simulink model "Funcion_de_Costo"  (R2018b)
settings: Solver=VariableStepAuto  StartTime=0.0  StopTime=10.0  RelTol=1e-3
undefined symbols (not defined in the file or in its folder): DiscIntNeverNeededParam
settings Model: Creator=of  LastModifiedBy=of

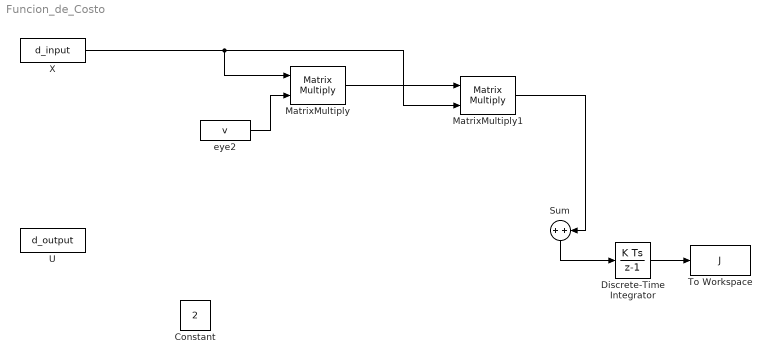
== system Funcion_de_Costo ==
  Constant : Constant  Value=2
  Discrete-Time Integrator : DiscreteIntegrator  SampleTime=-1  ICPrevOutput=DiscIntNeverNeededParam  ICPrevScaledInput=DiscIntNeverNeededParam
  MatrixMultiply : Product  Multiplication=Matrix(*)
  MatrixMultiply1 : Product  Multiplication=Matrix(*)
  Sum : Sum  Inputs=+|+
  To Workspace : ToWorkspace  VariableName=J  SaveFormat=Timeseries  SampleTime=-1
  U : FromWorkspace  VariableName=d_output  SampleTime=0
  X : FromWorkspace  VariableName=d_input  SampleTime=0
  "eye2 " : FromWorkspace  VariableName=v  SampleTime=0
  wires:
  MatrixMultiply/1 -> MatrixMultiply1/1
  X/1 -> MatrixMultiply/1, MatrixMultiply1/2
  Sum/1 -> Discrete-Time Integrator/1
  MatrixMultiply1/1 -> Sum/2
  Discrete-Time Integrator/1 -> To Workspace/1
  "eye2 "/1 -> MatrixMultiply/2
